simulink model "Template_obs_2019b_v2"  (R2019b)
settings: Solver=ode1  StartTime=0.0  StopTime=inf  FixedStep=0.002  RelTol=1e-3  EnableMultiTasking=on
PostLoadFcn:
  | qc_set_target_type(getConfigSet(bdroot, 'QUARC Default Target Configuration'));
values from neighbouring files (symbols this model uses):
  A_ob = A - L_kf*C    [LQ_KF_version1.m]    (also in LQ_KF_version2.m; LQ_Luenberger.m; PP_Luenberger.m = A - L*C; prova1.m = A - L*C)
  B_ob = [ B - L_kf*D, L_kf]    [LQ_KF_version1.m]    (also in LQ_KF_version2.m; LQ_Luenberger.m; PP_Luenberger.m = [ B, L]; prova1.m = [ B, L])
  C_ob = eye(n)    [LQ_KF_version1.m]    (also in LQ_KF_version2.m; LQ_Luenberger.m; PP_Luenberger.m; prova1.m)
  D_ob = zeros(n, m+p)    [LQ_KF_version1.m]    (also in LQ_KF_version2.m; LQ_Luenberger.m; PP_Luenberger.m; prova1.m)
  Ken_eta = K(:, 4)    [LQ_KF_version1.m]    (also in LQ_KF_version2.m = Ken(:, n+1:end); LQ_Luenberger.m; PP_Luenberger.m = Ken(:, n+1:end); prova1.m = Ken(:, n+1:end))
  Ken_x = K(:, 1:3)    [LQ_KF_version1.m]    (also in LQ_KF_version2.m = Ken(:, 1:n); LQ_Luenberger.m; PP_Luenberger.m = Ken(:, 1:n); prova1.m = Ken(:, 1:n))
undefined symbols (not defined in the file or in its folder): HIL, Kb, offset_corrente_volt, offset_posizione_volt, x1_eq0, x2_eq0
libraries: quarc_library x4, simulink x1
settings Model: SimulationMode=external  ExtModeTrigDuration=5000  Creator=CFulford  LastModifiedBy=Student
settings SolverCC: PositivePriorityOrder=on
settings DataIOCC: LimitDataPoints=on  SaveFormat=Array  SignalLoggingSaveFormat=ModelDataLogs  ReturnWorkspaceOutputs=off
settings OptimizationCC: ExpressionDepthLimit=2147483647  InitFltsAndDblsToZero=on  LifeSpan=inf
settings DebuggingCC: SaveWithParameterizedLinksMsg=none  UnderspecifiedInitializationDetection=Classic  MergeDetectMultiDrivingBlocksExec=none  SolverPrmCheckMsg=warning  MultiTaskDSMMsg=warning  MultiTaskCondExecSysMsg=none  FcnCallInpInsideContextMsg=warning  StateNameClashWarn=warning  SFUnexpectedBacktrackingDiag=warning  SFNoUnconditionalDefaultTransitionDiag=warning  SFExecutionAtInitializationDiag=none  ArithmeticOperatorsInVariantConditions=warning
settings HardwareCC: ProdBitPerPointer=32  ProdBitPerSizeT=32  ProdBitPerPtrDiffT=32  ProdLargestAtomicFloat=None  ProdIntDivRoundTo=Undefined  ProdEndianess=Unspecified  ProdWordSize=32  ProdHWDeviceType=32-bit Generic
settings ModelReferenceCC: PropagateSignalLabelsOutOfModel=off
settings SFSimCC: SimUseLocalCustomCode=off  CustomCodeUndefinedFunction=UseInterfaceOnly
settings RTWCC: Description=QUARC Win64 Target  SystemTargetFile=quarc_win64.tlc  TemplateMakefile=quarc_default_tmf  RTWUseLocalCustomCode=off
settings CodeAppCC: StateflowObjectComments=on
settings STFCustomTargetCC: TargetPreCompLibLocation=C:\PROGRA~3\QUARC\lib\2019b\win64\release  ConcurrentExecutionCompliant=on  CombineOutputUpdateFcns=on  CPPClassGenCompliant=on  SystemTargetFile=quarc_win64.tlc
settings GRTTargetCC: TargetPreCompLibLocation=C:\PROGRA~3\QUARC\lib\2019b\win64\release  TargetLangStandard=C89/C90 (ANSI)  ParMdlRefBuildCompliant=off  CompOptLevelCompliant=off  MatFileLogging=off  UseToolchainInfoCompliant=off  ExtMode=on  ExtModeMexFile=quarc_comm
settings ConfigComp: CovMetricSettings=dw  CovSaveCumulativeToWorkspaceVar=on  CovSaveSingleToWorkspaceVar=on  CovExternalEMLEnable=off  CovSFcnEnable=off

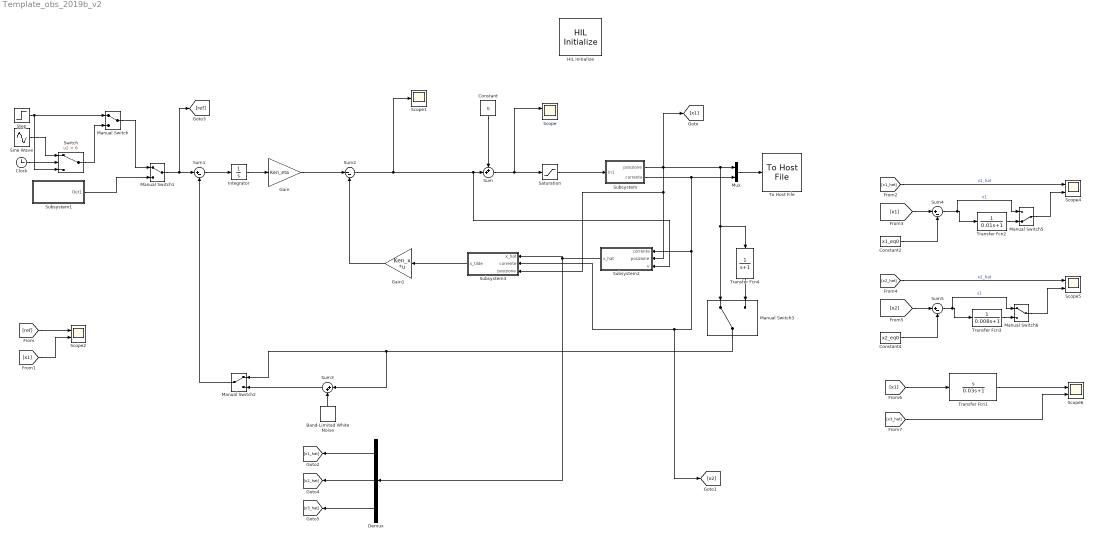
== system Template_obs_2019b_v2 ==
  Band-Limited White Noise : simulink/Sources/Band-Limited White Noise  Cov=[8.9934e-11*0.002]  Ts=0.002  seed=[23341]
  Clock : Clock
  Constant : Constant  Value=u
  Constant2 : Constant  Value=x1_eq0
  Constant4 : Constant  Value=x2_eq0
  Demux : Demux  Outputs=3
  Gain : Gain  Gain=Ken_eta
  Gain1 : Gain  Gain=Ken_x  Multiplication=Matrix(K*u) (u vector)
  HIL Initialize : quarc_library/Data Acquisition/Generic/Configuration/HIL Initialize  Priority=-99  object_name=HIL-1  board_type=q2_usb  board_number=0  board_options=d0=digital;d1=digital;led=auto;update_rate=normal;decimation=1  exclusive=off  active=off  hardware_clocks=[0]  clock_modes=[]  initial_clock_frequencies=[]  set_clock_params_at_start=off  set_clock_params_at_switch_in=off  set_clock_frequencies_at_start=off  set_clock_frequencies_at_switch_in=off  analog_input_channels=[0:1]  analog_input_configurations=[]  analog_input_maximums=10  analog_input_minimums=-10  set_analog_input_params_at_start=on  set_analog_input_params_at_switch_in=off  analog_output_channels=[0:1]  analog_output_maximums=10  analog_output_minimums=-10  initial_analog_outputs=[0]  final_analog_outputs=[0]  watchdog_analog_outputs=0  set_analog_output_params_at_start=on  set_analog_output_params_at_switch_in=off  set_analog_outputs_at_start=on  set_analog_outputs_at_switch_in=off  set_analog_outputs_at_terminate=on  set_analog_outputs_at_switch_out=off  set_analog_outputs_on_watchdog=off  digital_input_channels=[]  digital_output_channels=[]  digital_output_configuration=[]  initial_digital_outputs=[1]  final_digital_outputs=[1]  watchdog_digital_outputs=[1]  set_digital_output_params_at_start=off  set_digital_output_params_at_switch_in=off  set_digital_outputs_at_start=on  set_digital_outputs_at_switch_in=off  set_digital_outputs_at_terminate=on  set_digital_outputs_at_switch_out=off  set_digital_outputs_on_watchdog=off  encoder_channels=[0:1]  quadrature=[4]  encoder_filter_frequency=[]  initial_encoder_counts=[0]  set_encoder_params_at_start=on  set_encoder_params_at_switch_in=off  set_encoder_counts_at_start=on  set_encoder_counts_at_switch_in=off  pwm_channels=[]  pwm_modes=[0]  pwm_frequency=1/0.020  pwm_configuration=[]  pwm_alignment=[]  pwm_polarity=[]  pwm_leading_deadband=[]  pwm_trailing_deadband=[]  initial_pwm_outputs=[0]  final_pwm_outputs=[0]  watchdog_pwm_outputs=[0]  set_pwm_params_at_start=on  set_pwm_params_at_switch_in=off  set_pwm_outputs_at_start=on  set_pwm_outputs_at_switch_in=off  set_pwm_outputs_at_terminate=on  set_pwm_outputs_at_switch_out=off  set_pwm_outputs_on_watchdog=off  other_output_channels=[]  initial_other_outputs=[]  final_other_outputs=[]  watchdog_other_outputs=[]  set_other_outputs_at_start=off  set_other_outputs_at_switch_in=off  set_other_outputs_at_terminate=off  set_other_outputs_at_switch_out=off  set_other_outputs_on_watchdog=off
  Integrator : Integrator
  Manual Switch{,1..3,6} (5 alike) : ManualSwitch
  Manual Switch5 : ManualSwitch  CurrentSetting=0
  Mux : Mux  Inputs=2
  Saturation : Saturate  UpperLimit=23  LowerLimit=0
  Scope{,2,4..6} (5 alike) : Scope  NumInputPorts=2
  Scope1 : Scope
  Sine Wave : Sin  Amplitude=0.0005  Bias=0.004  SampleTime=0.002
  Step : Step  After=0.004  SampleTime=0.002
  Subsystem : Subsystem
  Subsystem1 : Subsystem
  Subsystem2 : Subsystem
  Subsystem3 : Subsystem
  Sum : Sum  Inputs=++|
  Sum1 : Sum  Inputs=|+-
  Sum2 : Sum  Inputs=|--
  Sum3 : Sum  Inputs=|++
  Sum4 : Sum  Inputs=|+-
  Sum5 : Sum  Inputs=|+-
  Switch : Switch  Criteria=u2 > Threshold  Threshold=6
  To Host File : quarc_library/Sinks/To Host/To Host File  file_name=data_%{date}_%{time}.mat  variable_name=data_%{date}_%{time}  decimation=1  sample_time=-1  file_format=MAT-file v.5  options=No header or footer  append=off  final_file_name=data_23-May-2025_13-29-56.mat  bitrate=2000000
  Transfer Fcn1 : TransferFcn  Numerator=[1 0]  Denominator=[0.03 1]
  Transfer Fcn2 : TransferFcn  Denominator=[0.01 1]
  Transfer Fcn3 : TransferFcn  Denominator=[0.008 1]
  Transfer Fcn4 : TransferFcn  Denominator=[1 1]
  wires:
  Mux/1 -> To Host File/1
  Subsystem/2(corrente) -> Mux/2, Subsystem3/2(corrente), [x2], Subsystem2/1(corrente)
  Subsystem2/1(x_hat) -> Demux/1, Subsystem3/1(x_hat)
  Manual Switch1/1 -> [ref], Sum1/1
  Subsystem3/1(x_tilde) -> Gain1/1
  Saturation/1 -> Subsystem/1(In1)
  Subsystem1/1(Out1) -> Manual Switch1/2
  Step/1 -> Switch/3, Manual Switch/1
  Sum2/1 -> Scope1/1, Subsystem2/3(u), Sum/2
  Gain1/1 -> Sum2/2
  Gain/1 -> Sum2/1
  Switch/1 -> Manual Switch/2
  Manual Switch/1 -> Manual Switch1/1
  Integrator/1 -> Gain/1
  Manual Switch2/1 -> Sum1/2
  Sine Wave/1 -> Switch/1
  Sum/1 -> Scope/1, Saturation/1
  Clock/1 -> Switch/2
  Sum1/1 -> Integrator/1
  Constant/1 -> Sum/1
  Subsystem/1(posizione) -> [x1], Subsystem3/3(posizione), Subsystem2/2(posizione), Mux/1, Transfer Fcn4/1, Manual Switch3/1
  Manual Switch3/1 -> Sum3/1, Manual Switch2/1
  Band-Limited White Noise/1 -> Sum3/2
  Sum3/1 -> Manual Switch2/2
  Demux/2 -> [x2_hat]
  Demux/1 -> [x1_hat]
  Demux/3 -> [x3_hat]
  [ref] -> Scope2/1
  [x1] -> Scope2/2
  [x2_hat] -> Scope5/1  "x2_hat"
  Manual Switch6/1 -> Scope5/2
  Transfer Fcn3/1 -> Manual Switch6/2
  [x2] -> Sum5/1
  Transfer Fcn2/1 -> Manual Switch5/2
  [x1] -> Sum4/1
  Sum5/1 -> Manual Switch6/1, Transfer Fcn3/1  "x1"
  Constant2/1 -> Sum4/2
  Constant4/1 -> Sum5/2
  [x1] -> Transfer Fcn1/1
  [x3_hat] -> Scope6/2
  [x1_hat] -> Scope4/1  "x1_hat"
  Transfer Fcn1/1 -> Scope6/1
  Manual Switch5/1 -> Scope4/2
  Sum4/1 -> Manual Switch5/1, Transfer Fcn2/1  "x1"
  Transfer Fcn4/1 -> Manual Switch3/2

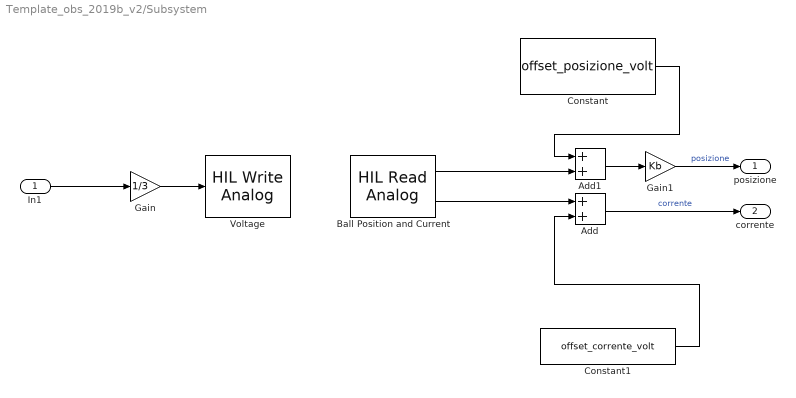
== system Template_obs_2019b_v2/Subsystem ==
  In1 : Inport
  Add : Sum
  Add1 : Sum
  Ball Position and Current : quarc_library/Data Acquisition/Generic/Immediate I//O/HIL Read Analog  object_name=HIL-1  channels=[0:1]  sample_time=qc_get_step_size  active=on  vector_output=off
  Constant : Constant  Value=offset_posizione_volt
  Constant1 : Constant  Value=offset_corrente_volt
  Gain : Gain  Gain=1/3
  Gain1 : Gain  Gain=Kb
  Voltage : quarc_library/Data Acquisition/Generic/Immediate I//O/HIL Write Analog  object_name=HIL-1  channels=0  sample_time=-1  active=off  vector_input=off
  posizione : Outport
  corrente : Outport  Port=2
  wires:
  Ball Position and Current/1 -> Add1/2
  Gain1/1 -> posizione/1  "posizione"
  Ball Position and Current/2 -> Add/1
  Constant1/1 -> Add/2
  Gain/1 -> Voltage/1
  Constant/1 -> Add1/1
  Add1/1 -> Gain1/1
  Add/1 -> corrente/1  "corrente"
  In1/1 -> Gain/1

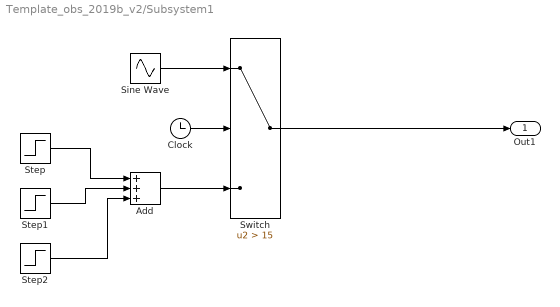
== system Template_obs_2019b_v2/Subsystem1 ==
  Add : Sum  Inputs=+++
  Clock : Clock
  Sine Wave : Sin  Amplitude=0.0015  Bias=0.005  SampleTime=0.002
  Step : Step  Time=3  After=0.003  SampleTime=0
  Step1 : Step  Time=5  After=0.006  SampleTime=0
  Step2 : Step  Time=10  After=-0.002  SampleTime=0
  Switch : Switch  Criteria=u2 > Threshold  Threshold=15
  Out1 : Outport
  wires:
  Switch/1 -> Out1/1
  Step/1 -> Add/1
  Step1/1 -> Add/2
  Step2/1 -> Add/3
  Add/1 -> Switch/3
  Clock/1 -> Switch/2
  Sine Wave/1 -> Switch/1

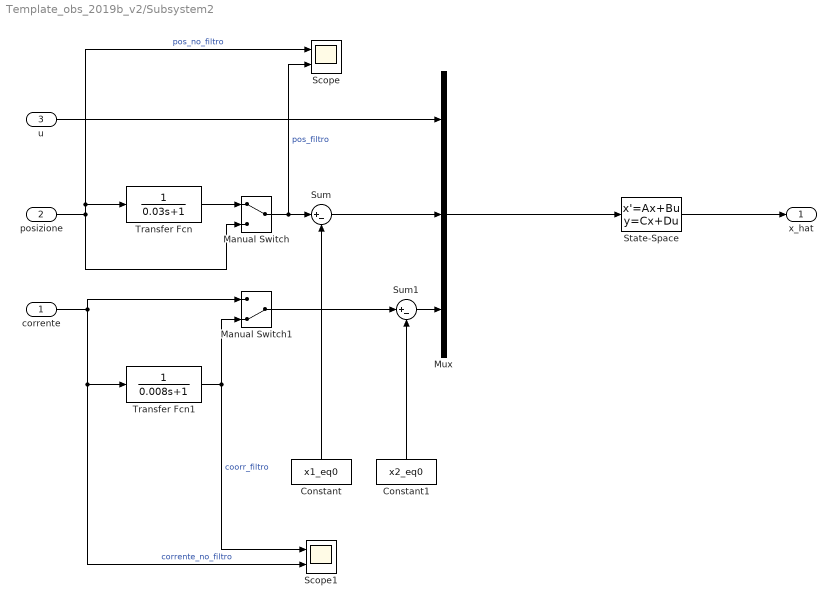
== system Template_obs_2019b_v2/Subsystem2 ==
  corrente : Inport
  posizione : Inport  Port=2
  u : Inport  Port=3
  Constant : Constant  Value=x1_eq0
  Constant1 : Constant  Value=x2_eq0
  Manual Switch : ManualSwitch
  Manual Switch1 : ManualSwitch  CurrentSetting=0
  Mux : Mux  Inputs=3
  Scope : Scope  NumInputPorts=2
  Scope1 : Scope  NumInputPorts=2
  State-Space : StateSpace  A=A_ob  B=B_ob  C=C_ob  D=D_ob  InitialCondition=[-x1_eq0, -x2_eq0, 0]
  Sum : Sum  Inputs=|+-
  Sum1 : Sum  Inputs=|+-
  Transfer Fcn : TransferFcn  Denominator=[0.03 1]
  Transfer Fcn1 : TransferFcn  Denominator=[0.008 1]
  x_hat : Outport
  wires:
  Constant/1 -> Sum/2
  Constant1/1 -> Sum1/2
  u/1 -> Mux/1
  Sum/1 -> Mux/2
  Sum1/1 -> Mux/3
  State-Space/1 -> x_hat/1
  Mux/1 -> State-Space/1
  Manual Switch/1 -> Scope/2, Sum/1  "pos_filtro"
  posizione/1 -> Scope/1, Transfer Fcn/1, Manual Switch/2  "pos_no_filtro"
  Transfer Fcn/1 -> Manual Switch/1
  Manual Switch1/1 -> Sum1/1
  corrente/1 -> Scope1/2, Transfer Fcn1/1, Manual Switch1/1  "corrente_no_filtro"
  Transfer Fcn1/1 -> Scope1/1, Manual Switch1/2  "coorr_filtro"

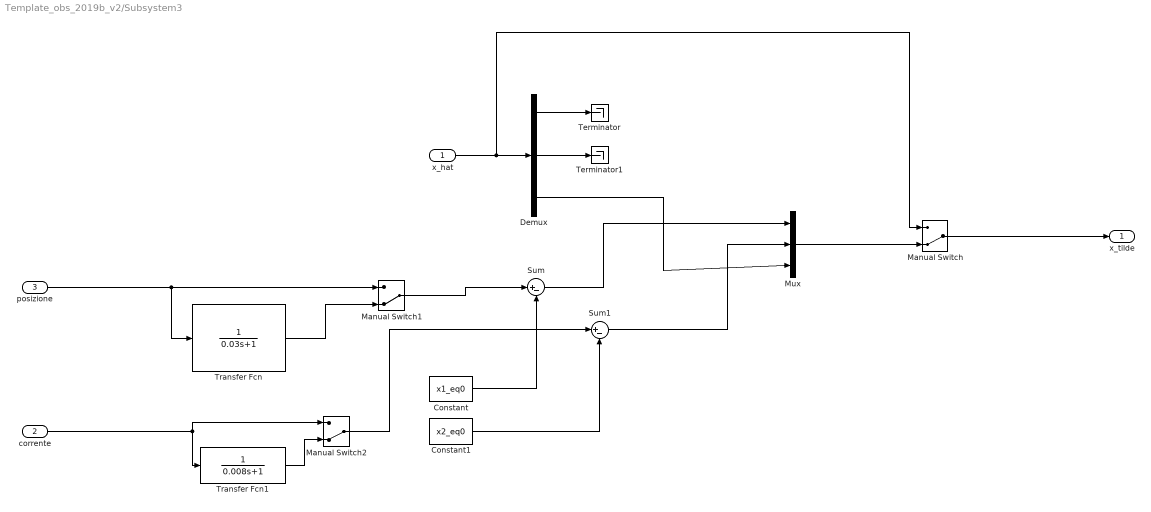
== system Template_obs_2019b_v2/Subsystem3 ==
  x_hat : Inport
  corrente : Inport  Port=2
  posizione : Inport  Port=3
  Constant : Constant  Value=x1_eq0
  Constant1 : Constant  Value=x2_eq0
  Demux : Demux  Outputs=3
  Manual Switch : ManualSwitch  CurrentSetting=0
  Manual Switch1 : ManualSwitch  CurrentSetting=0
  Manual Switch2 : ManualSwitch  CurrentSetting=0
  Mux : Mux  Inputs=3
  Sum : Sum  Inputs=|+-
  Sum1 : Sum  Inputs=|+-
  Terminator : Terminator
  Terminator1 : Terminator
  Transfer Fcn : TransferFcn  Denominator=[0.03 1]
  Transfer Fcn1 : TransferFcn  Denominator=[0.008 1]
  x_tilde : Outport
  wires:
  x_hat/1 -> Manual Switch/1, Demux/1
  Manual Switch/1 -> x_tilde/1
  Demux/1 -> Terminator/1
  Demux/2 -> Terminator1/1
  Mux/1 -> Manual Switch/2
  Demux/3 -> Mux/3
  Sum/1 -> Mux/1
  Sum1/1 -> Mux/2
  Constant/1 -> Sum/2
  Constant1/1 -> Sum1/2
  posizione/1 -> Manual Switch1/1, Transfer Fcn/1
  Manual Switch1/1 -> Sum/1
  Transfer Fcn/1 -> Manual Switch1/2
  corrente/1 -> Transfer Fcn1/1, Manual Switch2/1
  Manual Switch2/1 -> Sum1/1
  Transfer Fcn1/1 -> Manual Switch2/2
